simulink model "nonlinear_simulation_tracking"  (R2023a)
settings: Solver=VariableStepAuto  StartTime=0.0  StopTime=10.0  RelTol=1e-3
model workspace: external: MATLAB File C:\Uni\Projektarbeit\matlab\nonlinear_fo_prep.m (data not in the file)
undefined symbols (not defined in the file): init_cond
libraries: simulink x2
settings Model: Creator=morit  LastModifiedBy=morit

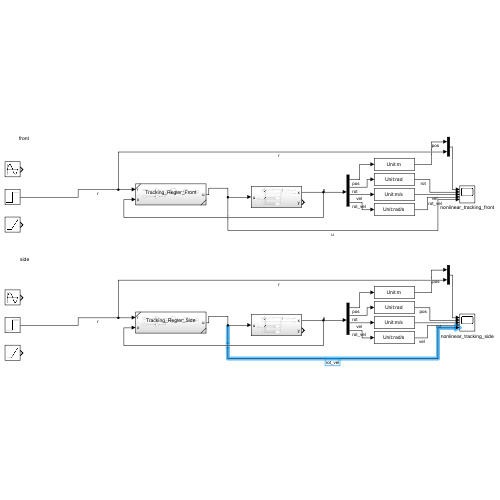
[thumbnail: Simulink's stored preview of the top-level diagram]
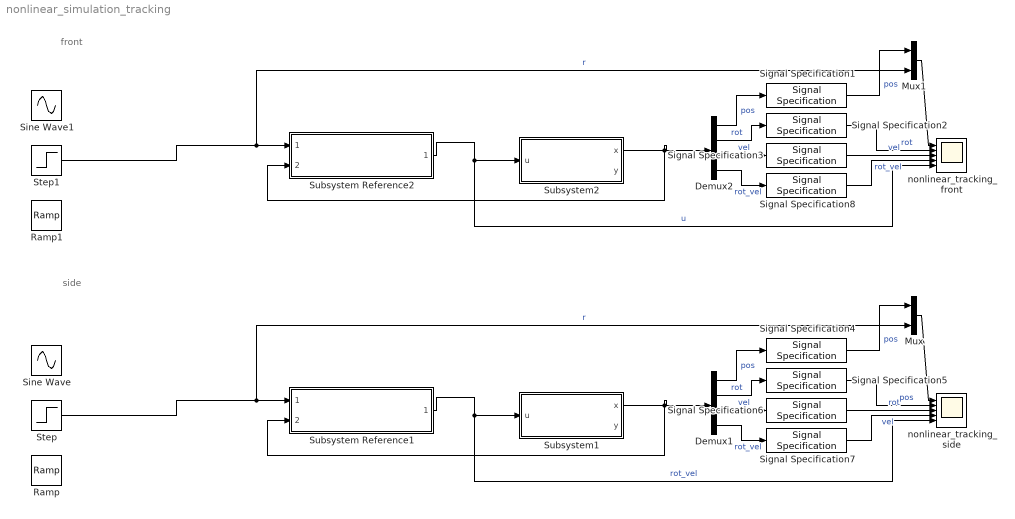
== system nonlinear_simulation_tracking ==
  note: side
  note: front
  Demux1 : Demux
  Demux2 : Demux
  Mux : Mux  Inputs=2
  Mux1 : Mux  Inputs=2
  Ramp : simulink/Sources/Ramp  slope=0.01  start=0  InitialOutput=0
  Ramp1 : simulink/Sources/Ramp  slope=0.01  start=0  InitialOutput=0
  Signal Specification1 : SignalSpecification  Unit=m
  Signal Specification2 : SignalSpecification  Unit=rad
  Signal Specification3 : SignalSpecification  Unit=m/s
  Signal Specification4 : SignalSpecification  Unit=m
  Signal Specification5 : SignalSpecification  Unit=rad
  Signal Specification6 : SignalSpecification  Unit=m/s
  Signal Specification7 : SignalSpecification  Unit=rad/s
  Signal Specification8 : SignalSpecification  Unit=rad/s
  Sine Wave : Sin  Amplitude=0.05  Frequency=0.3  SampleTime=0
  Sine Wave1 : Sin  Amplitude=0.05  Frequency=0.3  SampleTime=0
  Step : Step  After=0.05  SampleTime=0
  Step1 : Step  After=0.05  SampleTime=0
  Subsystem Reference1 : Subsystem  ReferencedSubsystem=Tracking_Regler_Side
  Subsystem Reference2 : Subsystem  ReferencedSubsystem=Tracking_Regler_Front
  Subsystem1 : Subsystem
  Subsystem2 : Subsystem
  nonlinear_tracking_front : Scope  NumInputPorts=5
  nonlinear_tracking_side : Scope  NumInputPorts=5
  wires:
  Signal Specification6/1 -> nonlinear_tracking_side/3  "rot"
  Subsystem Reference1/1 -> nonlinear_tracking_side/5, Subsystem1/1(u)  "rot_vel"
  Signal Specification5/1 -> nonlinear_tracking_side/2  "pos"
  Demux1/1 -> Signal Specification4/1  "pos"
  Demux1/4 -> Signal Specification7/1  "rot_vel"
  Demux1/3 -> Signal Specification6/1  "vel"
  Demux1/2 -> Signal Specification5/1  "rot"
  Subsystem1/1(x) -> Demux1/1, Subsystem Reference1/2
  Signal Specification7/1 -> nonlinear_tracking_side/4  "vel"
  Step/1 -> Mux/2, Subsystem Reference1/1  "r"
  Mux/1 -> nonlinear_tracking_side/1
  Signal Specification4/1 -> Mux/1  "pos"
  Subsystem Reference2/1 -> nonlinear_tracking_front/5, Subsystem2/1(u)  "u"
  Demux2/4 -> Signal Specification8/1  "rot_vel"
  Signal Specification8/1 -> nonlinear_tracking_front/4  "rot_vel"
  Signal Specification3/1 -> nonlinear_tracking_front/3  "vel"
  Signal Specification1/1 -> Mux1/1  "pos"
  Mux1/1 -> nonlinear_tracking_front/1
  Step1/1 -> Mux1/2, Subsystem Reference2/1  "r"
  Demux2/1 -> Signal Specification1/1  "pos"
  Subsystem2/1(x) -> Demux2/1, Subsystem Reference2/2
  Demux2/3 -> Signal Specification3/1  "vel"
  Signal Specification2/1 -> nonlinear_tracking_front/2  "rot"
  Demux2/2 -> Signal Specification2/1  "rot"

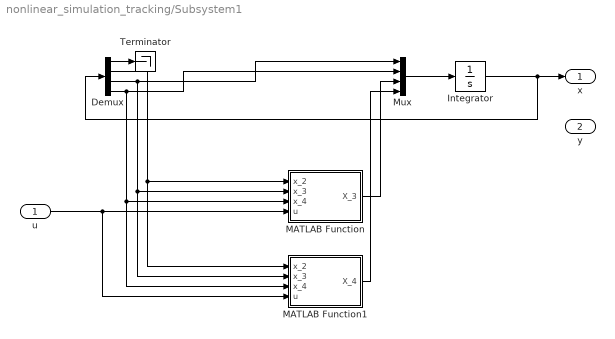
== system nonlinear_simulation_tracking/Subsystem1 ==
  u : Inport
  Demux : Demux
  Integrator : Integrator  InitialCondition=init_cond
  MATLAB Function : MATLAB Function  TreatAsAtomicUnit=on
  MATLAB Function1 : MATLAB Function  TreatAsAtomicUnit=on
  Mux : Mux
  Terminator : Terminator
  x : Outport
  y : Outport  Port=2
  wires:
  u/1 -> MATLAB Function1/4(u), MATLAB Function/4(u)
  Integrator/1 -> Demux/1, x/1
  Mux/1 -> Integrator/1
  Demux/3 -> MATLAB Function1/2(x_3), MATLAB Function/2(x_3), Mux/1
  Demux/4 -> MATLAB Function1/3(x_4), MATLAB Function/3(x_4), Mux/2
  Demux/2 -> MATLAB Function1/1(x_2), MATLAB Function/1(x_2)
  MATLAB Function/1(X_3) -> Mux/3
  MATLAB Function1/1(X_4) -> Mux/4
  Demux/1 -> Terminator/1

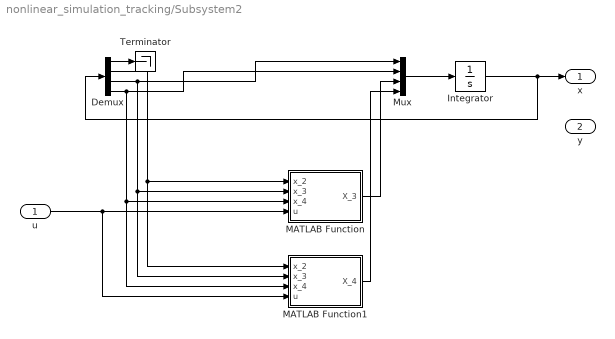
== system nonlinear_simulation_tracking/Subsystem2 ==
  u : Inport
  Demux : Demux
  Integrator : Integrator  InitialCondition=init_cond
  MATLAB Function : MATLAB Function  TreatAsAtomicUnit=on
  MATLAB Function1 : MATLAB Function  TreatAsAtomicUnit=on
  Mux : Mux
  Terminator : Terminator
  x : Outport
  y : Outport  Port=2
  wires:
  u/1 -> MATLAB Function1/4(u), MATLAB Function/4(u)
  Integrator/1 -> Demux/1, x/1
  Mux/1 -> Integrator/1
  Demux/3 -> MATLAB Function1/2(x_3), MATLAB Function/2(x_3), Mux/1
  Demux/4 -> MATLAB Function1/3(x_4), MATLAB Function/3(x_4), Mux/2
  Demux/2 -> MATLAB Function1/1(x_2), MATLAB Function/1(x_2)
  MATLAB Function/1(X_3) -> Mux/3
  MATLAB Function1/1(X_4) -> Mux/4
  Demux/1 -> Terminator/1

== matlab function nonlinear_simulation_tracking/Subsystem2/MATLAB Function ==
  data: x_2 input; x_3 input; x_4 input; u input; X_3 output
function X_3 = fcn(x_2, x_3, x_4, u)

X_3 = (0.25932*(0.00033747*sin(x_2)*x_4^2 + 0.2304*x_3 - 0.012024*u + 0.017424*cos(x_2)*sin(x_2)))/(0.00046059*cos(x_2)^2 - 0.00047314);

== matlab function nonlinear_simulation_tracking/Subsystem2/MATLAB Function1 ==
  data: x_2 input; x_3 input; x_4 input; u input; X_4 output
function X_4 = fcn(x_2, x_3, x_4, u)

X_4 = -(54.484*(8.4536e-6*cos(x_2)*sin(x_2)*x_4^2 + 0.00044837*sin(x_2) + 0.012024*cos(x_2)*(0.48*x_3 - 0.02505*u)))/(0.00046059*cos(x_2)^2 - 0.00047314);

== matlab function nonlinear_simulation_tracking/Subsystem1/MATLAB Function ==
  data: x_2 input; x_3 input; x_4 input; u input; X_3 output
function X_3 = fcn(x_2, x_3, x_4, u)

X_3 = (0.25932*(0.00033747*sin(x_2)*x_4^2 + 0.2304*x_3 - 0.012024*u + 0.017424*cos(x_2)*sin(x_2)))/(0.00046059*cos(x_2)^2 - 0.00047314);

== matlab function nonlinear_simulation_tracking/Subsystem1/MATLAB Function1 ==
  data: x_2 input; x_3 input; x_4 input; u input; X_4 output
function X_4 = fcn(x_2, x_3, x_4, u)

X_4 = -(54.484*(8.4536e-6*cos(x_2)*sin(x_2)*x_4^2 + 0.00044837*sin(x_2) + 0.012024*cos(x_2)*(0.48*x_3 - 0.02505*u)))/(0.00046059*cos(x_2)^2 - 0.00047314);
